simulink model "StateObserverTest1"  (R2018b)
settings: Solver=VariableStepAuto  StartTime=0.0  StopTime=90  RelTol=1e-3
values from neighbouring files (symbols this model uses):
  GdSpeed = c2d(Gspeed,Ts,'tustin')    [DiscreteObserverAndSFB.m]
  K = -lqrd (Aaugmented,Baugmented,Qespeed,Respeed,Ts)    [DiscreteObserverAndSFB.m]
  Ltr = L'    [DiscreteObserverAndSFB.m]
  Ts = 0.01    [DiscreteObserverAndSFB.m]
undefined symbols (not defined in the file or in its folder): DiscIntNeverNeededParam
settings Model: Creator=mmbio  LastModifiedBy=mmbio

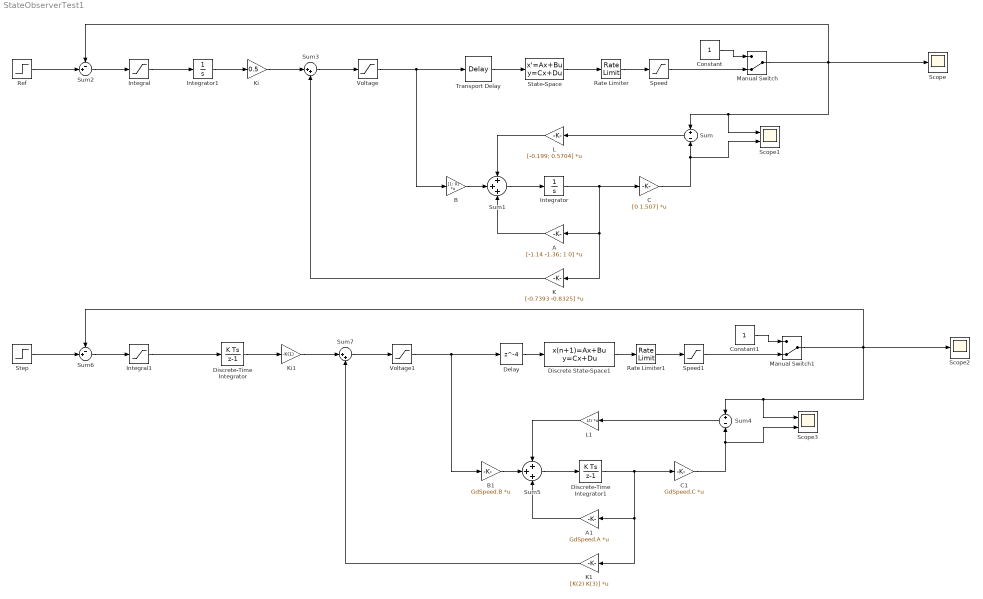
== system StateObserverTest1 ==
  A : Gain  Gain=[-1.14 -1.36; 1 0]  Multiplication=Matrix(K*u)
  A1 : Gain  Gain=GdSpeed.A  Multiplication=Matrix(K*u)
  B : Gain  Gain=[1; 0]  Multiplication=Matrix(K*u)
  B1 : Gain  Gain=GdSpeed.B  Multiplication=Matrix(K*u)
  C : Gain  Gain=[0 1.507]  Multiplication=Matrix(K*u)
  C1 : Gain  Gain=GdSpeed.C  Multiplication=Matrix(K*u)
  Constant : Constant
  Constant1 : Constant
  Delay : Delay  DelayLength=4  SampleTime=Ts
  Discrete State-Space1 : DiscreteStateSpace  A=GdSpeed.A  B=GdSpeed.B  C=GdSpeed.C  D=0  SampleTime=Ts
  Discrete-Time Integrator : DiscreteIntegrator  SampleTime=Ts  ICPrevOutput=DiscIntNeverNeededParam  ICPrevScaledInput=DiscIntNeverNeededParam
  Discrete-Time Integrator1 : DiscreteIntegrator  SampleTime=Ts  ICPrevOutput=DiscIntNeverNeededParam  ICPrevScaledInput=DiscIntNeverNeededParam
  Integral : Saturate  UpperLimit=5/0.5  LowerLimit=-5/0.5
  Integral1 : Saturate  UpperLimit=5/0.5  LowerLimit=-5/0.5
  Integrator : Integrator
  Integrator1 : Integrator
  K : Gain  Gain=[-0.7393 -0.8325]  Multiplication=Matrix(K*u)
  K1 : Gain  Gain=[K(2) K(3)]  Multiplication=Matrix(K*u)
  Ki : Gain  Gain=0.5
  Ki1 : Gain  Gain=-K(1)
  L : Gain  Gain=[-0.199; 0.5704]  Multiplication=Matrix(K*u)
  L1 : Gain  Gain=Ltr  Multiplication=Matrix(K*u)
  Manual Switch : ManualSwitch  CurrentSetting=0
  Manual Switch1 : ManualSwitch  CurrentSetting=0
  Rate Limiter : RateLimiter  RisingSlewLimit=0.65  FallingSlewLimit=-0.65  SampleTimeMode=inherited
  Rate Limiter1 : RateLimiter  RisingSlewLimit=0.65  FallingSlewLimit=-0.65  SampleTimeMode=inherited
  Ref : Step  SampleTime=0
  Scope : Scope
  Scope1 : Scope  NumInputPorts=2
  Scope2 : Scope
  Scope3 : Scope  NumInputPorts=2
  Speed : Saturate  UpperLimit=1000  LowerLimit=0
  Speed1 : Saturate  UpperLimit=1000  LowerLimit=0
  State-Space : StateSpace  A=[-1.14 -1.36; 1 0]  B=[1; 0]  C=[0.0 1.507]  D=0  InitialCondition=0
  Step : Step  SampleTime=0
  Sum : Sum  Inputs=+-
  Sum1 : Sum  Inputs=+++
  Sum2 : Sum  Inputs=-+|
  Sum3 : Sum  Inputs=|++
  Sum4 : Sum  Inputs=+-
  Sum5 : Sum  Inputs=+++
  Sum6 : Sum  Inputs=-+|
  Sum7 : Sum  Inputs=|++
  Transport Delay : TransportDelay  DelayTime=0.45
  Voltage : Saturate  UpperLimit=5  LowerLimit=0
  Voltage1 : Saturate  UpperLimit=5  LowerLimit=0
  wires:
  State-Space/1 -> Rate Limiter/1
  C/1 -> Scope1/2, Sum/2
  Sum/1 -> L/1
  Sum1/1 -> Integrator/1
  L/1 -> Sum1/1
  Integrator/1 -> K/1, A/1, C/1
  A/1 -> Sum1/3
  Sum2/1 -> Integral/1
  Ref/1 -> Sum2/2
  Integrator1/1 -> Ki/1
  K/1 -> Sum3/2
  B/1 -> Sum1/2
  Ki/1 -> Sum3/1
  Transport Delay/1 -> State-Space/1
  Rate Limiter/1 -> Speed/1
  Voltage/1 -> Transport Delay/1, B/1
  Sum3/1 -> Voltage/1
  Manual Switch/1 -> Sum/1, Scope1/1, Scope/1, Sum2/1
  Speed/1 -> Manual Switch/2
  Constant/1 -> Manual Switch/1
  L1/1 -> Sum5/1
  Sum7/1 -> Voltage1/1
  K1/1 -> Sum7/2
  Discrete-Time Integrator/1 -> Ki1/1
  A1/1 -> Sum5/3
  Discrete-Time Integrator1/1 -> K1/1, A1/1, C1/1
  Rate Limiter1/1 -> Speed1/1
  C1/1 -> Scope3/2, Sum4/2
  B1/1 -> Sum5/2
  Voltage1/1 -> Delay/1, B1/1
  Ki1/1 -> Sum7/1
  Step/1 -> Sum6/2
  Sum4/1 -> L1/1
  Sum6/1 -> Integral1/1
  Speed1/1 -> Manual Switch1/2
  Constant1/1 -> Manual Switch1/1
  Manual Switch1/1 -> Scope2/1, Scope3/1, Sum4/1, Sum6/1
  Sum5/1 -> Discrete-Time Integrator1/1
  Discrete State-Space1/1 -> Rate Limiter1/1
  Delay/1 -> Discrete State-Space1/1
  Integral/1 -> Integrator1/1
  Integral1/1 -> Discrete-Time Integrator/1
